simulink model "ExampleTransformation"  (R2024a)
settings: Solver=FixedStepAuto  StartTime=0.0  StopTime=inf  FixedStep=0.02  RelTol=1e-3  EnableMultiTasking=on
undefined symbols (not defined in the file): atmosphericScattering, basicProperties, castShadow, emissionColorMultiplier, meshID, position, quaternion, scale, visible
libraries: PRISMA x17, simulink_extras x3, GenericTarget x1
settings Model: Creator=damerius  LastModifiedBy=Scythe
settings SolverCC: ConcurrentTasks=on  AlgebraicLoopSolver=TrustRegion  PositivePriorityOrder=on
settings DataIOCC: SaveOutput=off  SignalLogging=off  DSMLogging=off  SaveTime=off  ReturnWorkspaceOutputs=off
settings OptimizationCC: DefaultParameterBehavior=Inlined  ReuseModelBlockBuffer=off  ZeroExternalMemoryAtStartup=off  ZeroInternalMemoryAtStartup=off  SimCompilerOptimization=on
settings DebuggingCC: UnconnectedInputMsg=warning  UnconnectedOutputMsg=warning  UnconnectedLineMsg=warning
settings HardwareCC: ProdBitPerLong=64  ProdHWDeviceType=Intel->x86-64 (Linux 64)
settings ModelReferenceCC: EnableRefExpFcnMdlSchedulingChecks=on
settings SFSimCC: SimParseCustomCode=off  SimGenImportedTypeDefs=on  SimTargetLang=C++
settings RTWCC: GenCodeOnly=on  PackageGeneratedCodeAndArtifacts=on  PackageName=PackNGo  RTWVerbose=off  BuildConfiguration=Faster Runs  TargetLang=C++  GPUComputeCapability=3.5  DLArmComputeVersion=19.05
settings CodeAppCC: ForceParamTrailComments=on  MaxIdLength=95  MATLABSourceComments=on  UseSimReservedNames=on
settings GRTTargetCC: TargetLangStandard=C++11 (ISO)  GenerateFullHeader=off  MatFileLogging=off  CodeInterfacePackaging=C++ class

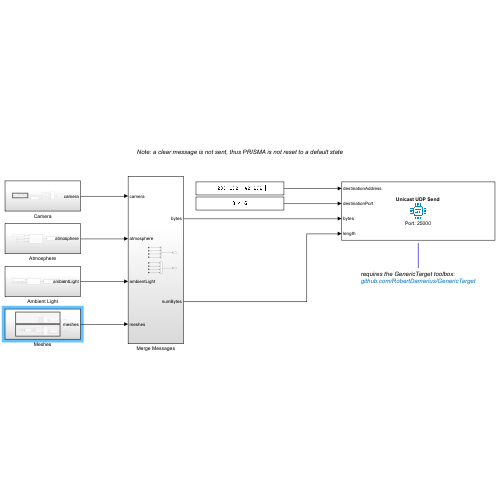
[thumbnail: Simulink's stored preview of the top-level diagram]
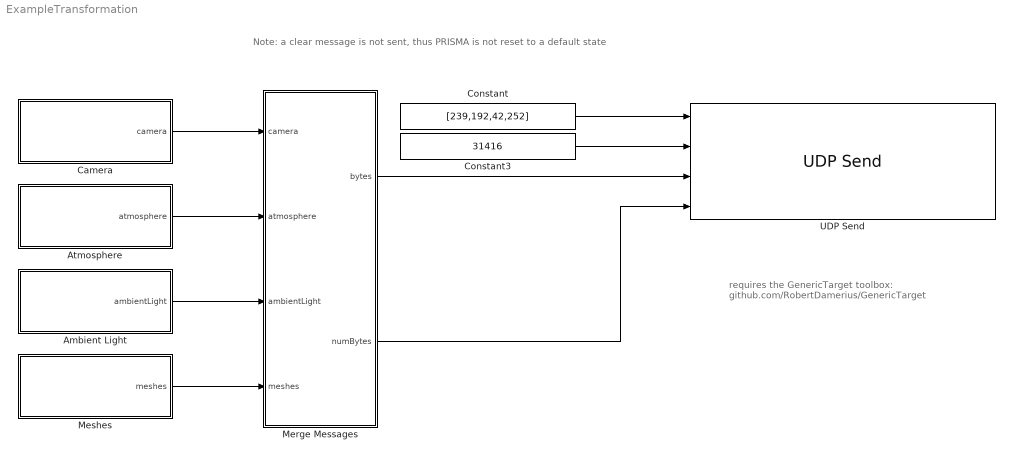
== system ExampleTransformation ==
  note: Note: a clear message is not sent, thus PRISMA is not reset to a default state
  note: requires the GenericTarget toolbox:
      | github.com/RobertDamerius/GenericTarget
  Ambient Light : Subsystem
  Atmosphere : Subsystem
  Camera : Subsystem
  Constant : Constant  Value=[239,192,42,252]  OutDataTypeStr=uint8
  Constant3 : Constant  Value=31416  OutDataTypeStr=uint16
  Merge Messages : Subsystem
  Meshes : Subsystem
  UDP Send : GenericTarget/Interface/UDP Send  showDetails=off  interfacePort=25000  interfaceIP=[0,0,0,0]  deviceName=''  prioritySocket=6  allowBroadcast=off  SampleTime=-1
      settings: SourceProductName=Generic Target
  wires:
  Constant3/1 -> UDP Send/2
  Camera/1(camera) -> Merge Messages/1(camera)
  Meshes/1(meshes) -> Merge Messages/4(meshes)
  Merge Messages/1(bytes) -> UDP Send/3
  Merge Messages/2(numBytes) -> UDP Send/4
  Ambient Light/1(ambientLight) -> Merge Messages/3(ambientLight)
  Constant/1 -> UDP Send/1
  Atmosphere/1(atmosphere) -> Merge Messages/2(atmosphere)

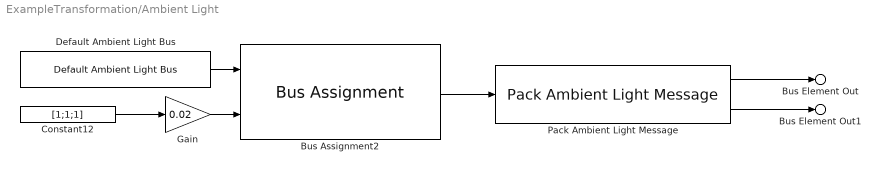
== system ExampleTransformation/Ambient Light ==
  Bus Assignment2 : BusAssignment  AssignedSignals=color
  Constant12 : Constant  Value=[1;1;1]
  Default Ambient Light Bus : PRISMA/Default Ambient Light Bus
      settings: SourceProductName=PRISMA
  Gain : Gain  Gain=0.02
  Pack Ambient Light Message : PRISMA/Pack Ambient Light Message
      settings: SourceProductName=PRISMA
  Bus Element Out : Outport  PortName=ambientLight  Element=bytes
  Bus Element Out1 : Outport  PortName=ambientLight  Element=numBytes
  wires:
  Pack Ambient Light Message/2 -> Bus Element Out1/1
  Pack Ambient Light Message/1 -> Bus Element Out/1
  Gain/1 -> Bus Assignment2/2
  Constant12/1 -> Gain/1
  Default Ambient Light Bus/1 -> Bus Assignment2/1
  Bus Assignment2/1 -> Pack Ambient Light Message/1

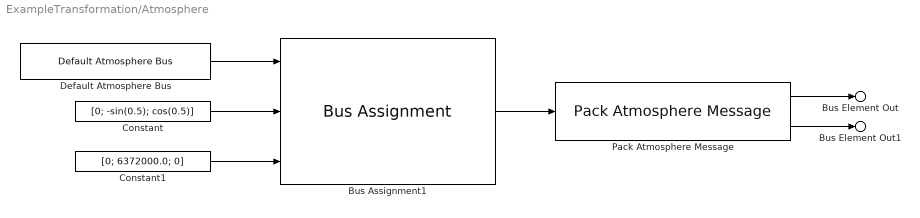
== system ExampleTransformation/Atmosphere ==
  Bus Assignment1 : BusAssignment  AssignedSignals=basicProperties.sunLightDirection,atmosphericScattering.eyePosition
  Constant : Constant  Value=[0; -sin(0.5); cos(0.5)]
  Constant1 : Constant  Value=[0; 6372000.0; 0]
  Default Atmosphere Bus : PRISMA/Default Atmosphere Bus
      settings: SourceProductName=PRISMA
  Pack Atmosphere Message : PRISMA/Pack Atmosphere Message
      settings: SourceProductName=PRISMA
  Bus Element Out : Outport  PortName=atmosphere  Element=bytes
  Bus Element Out1 : Outport  PortName=atmosphere  Element=numBytes
  wires:
  Bus Assignment1/1 -> Pack Atmosphere Message/1
  Default Atmosphere Bus/1 -> Bus Assignment1/1
  Pack Atmosphere Message/1 -> Bus Element Out/1
  Pack Atmosphere Message/2 -> Bus Element Out1/1
  Constant/1 -> Bus Assignment1/2
  Constant1/1 -> Bus Assignment1/3

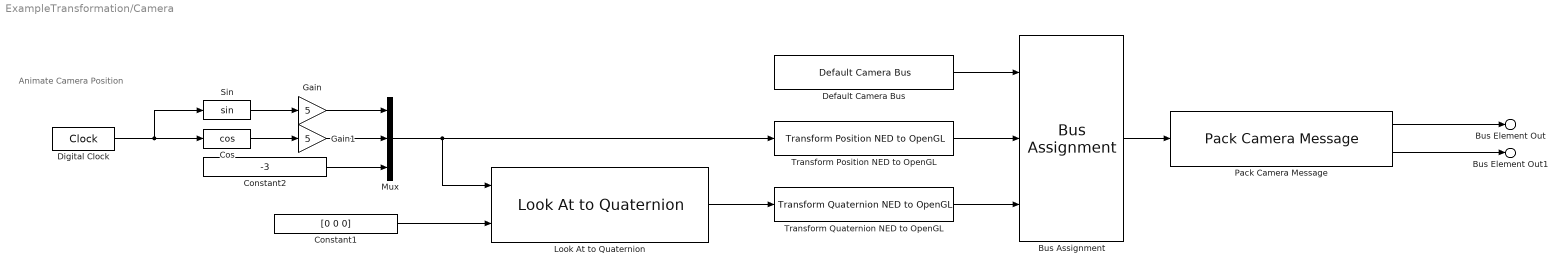
== system ExampleTransformation/Camera ==
  note: Animate Camera Position
  Bus Assignment : BusAssignment  AssignedSignals=position,quaternion
  Constant1 : Constant  Value=[0 0 0]
  Constant2 : Constant  Value=-3
  Cos : Trigonometry  Operator=cos
  Default Camera Bus : PRISMA/Default Camera Bus
      settings: SourceProductName=PRISMA
  Digital Clock : DigitalClock  SampleTime=0.02
  Gain : Gain  Gain=5
  Gain1 : Gain  Gain=5
  Look At to Quaternion : PRISMA/Transformation/Look At to Quaternion
      settings: SourceProductName=PRISMA
  Mux : Mux  Inputs=3
  Pack Camera Message : PRISMA/Pack Camera Message
      settings: SourceProductName=PRISMA
  Sin : Trigonometry
  Transform Position NED to OpenGL : PRISMA/Transformation/Transform Position NED to OpenGL
      settings: SourceProductName=PRISMA
  Transform Quaternion NED to OpenGL : PRISMA/Transformation/Transform Quaternion NED to OpenGL
      settings: SourceProductName=PRISMA
  Bus Element Out : Outport  PortName=camera  Element=bytes
  Bus Element Out1 : Outport  PortName=camera  Element=numBytes
  wires:
  Default Camera Bus/1 -> Bus Assignment/1
  Bus Assignment/1 -> Pack Camera Message/1
  Transform Position NED to OpenGL/1 -> Bus Assignment/2
  Transform Quaternion NED to OpenGL/1 -> Bus Assignment/3
  Look At to Quaternion/1 -> Transform Quaternion NED to OpenGL/1
  Mux/1 -> Look At to Quaternion/1, Transform Position NED to OpenGL/1
  Constant1/1 -> Look At to Quaternion/2
  Pack Camera Message/1 -> Bus Element Out/1
  Pack Camera Message/2 -> Bus Element Out1/1
  Constant2/1 -> Mux/3
  Sin/1 -> Gain/1
  Gain/1 -> Mux/1
  Cos/1 -> Gain1/1
  Gain1/1 -> Mux/2
  Digital Clock/1 -> Sin/1, Cos/1

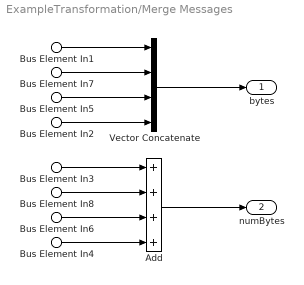
== system ExampleTransformation/Merge Messages ==
  Bus Element In1 : Inport  PortName=camera  Element=bytes
  Bus Element In3 : Inport  PortName=camera  Element=numBytes
  Bus Element In7 : Inport  Port=2  PortName=atmosphere  Element=bytes
  Bus Element In8 : Inport  Port=2  PortName=atmosphere  Element=numBytes
  Bus Element In5 : Inport  Port=3  PortName=ambientLight  Element=bytes
  Bus Element In6 : Inport  Port=3  PortName=ambientLight  Element=numBytes
  Bus Element In2 : Inport  Port=4  PortName=meshes  Element=bytes
  Bus Element In4 : Inport  Port=4  PortName=meshes  Element=numBytes
  Add : Sum  Inputs=++++
  Vector Concatenate : Concatenate  NumInputs=4
  bytes : Outport
  numBytes : Outport  Port=2
  wires:
  Bus Element In1/1 -> Vector Concatenate/1
  Bus Element In2/1 -> Vector Concatenate/4
  Bus Element In3/1 -> Add/1
  Bus Element In4/1 -> Add/4
  Vector Concatenate/1 -> bytes/1
  Add/1 -> numBytes/1
  Bus Element In5/1 -> Vector Concatenate/3
  Bus Element In6/1 -> Add/3
  Bus Element In7/1 -> Vector Concatenate/2
  Bus Element In8/1 -> Add/2

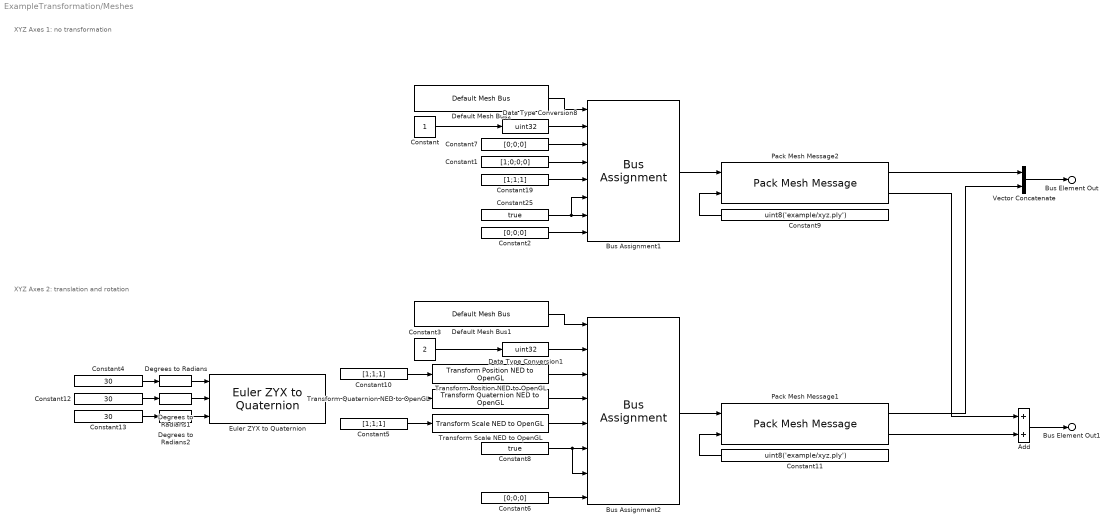
== system ExampleTransformation/Meshes ==
  note: XYZ Axes 1: no transformation
  note: XYZ Axes 2: translation and rotation
  Add : Sum
  Bus Assignment1 : BusAssignment  AssignedSignals=meshID,position,quaternion,scale,visible,castShadow,emissionColorMultiplier
  Bus Assignment2 : BusAssignment  AssignedSignals=meshID,position,quaternion,scale,visible,castShadow,emissionColorMultiplier
  Constant : Constant
  Constant1 : Constant  Value=[1;0;0;0]
  Constant10 : Constant  Value=[1;1;1]
  Constant11 : Constant  Value=uint8('example/xyz.ply')  OutDataTypeStr=uint8
  Constant12 : Constant  Value=30
  Constant13 : Constant  Value=30
  Constant19 : Constant  Value=[1;1;1]
  Constant2 : Constant  Value=[0;0;0]
  Constant25 : Constant  Value=true  OutDataTypeStr=boolean
  Constant3 : Constant  Value=2
  Constant4 : Constant  Value=30
  Constant5 : Constant  Value=[1;1;1]
  Constant6 : Constant  Value=[0;0;0]
  Constant7 : Constant  Value=[0;0;0]
  Constant8 : Constant  Value=true  OutDataTypeStr=boolean
  Constant9 : Constant  Value=uint8('example/xyz.ply')  OutDataTypeStr=uint8
  Data Type Conversion1 : DataTypeConversion  OutDataTypeStr=uint32  SaturateOnIntegerOverflow=off  RndMeth=Floor
  Data Type Conversion8 : DataTypeConversion  OutDataTypeStr=uint32  SaturateOnIntegerOverflow=off  RndMeth=Floor
  Default Mesh Bus1 : PRISMA/Default Mesh Bus
      settings: SourceProductName=PRISMA
  Default Mesh Bus2 : PRISMA/Default Mesh Bus
      settings: SourceProductName=PRISMA
  Degrees to Radians : simulink_extras/Transformations/Degrees to Radians
  Degrees to Radians1 : simulink_extras/Transformations/Degrees to Radians
  Degrees to Radians2 : simulink_extras/Transformations/Degrees to Radians
  Euler ZYX to Quaternion : PRISMA/Transformation/Euler ZYX to Quaternion
      settings: SourceProductName=PRISMA
  Pack Mesh Message1 : PRISMA/Pack Mesh Message
      settings: SourceProductName=PRISMA
  Pack Mesh Message2 : PRISMA/Pack Mesh Message
      settings: SourceProductName=PRISMA
  Transform Position NED to OpenGL : PRISMA/Transformation/Transform Position NED to OpenGL
      settings: SourceProductName=PRISMA
  Transform Quaternion NED to OpenGL : PRISMA/Transformation/Transform Quaternion NED to OpenGL
      settings: SourceProductName=PRISMA
  Transform Scale NED to OpenGL : PRISMA/Transformation/Transform Scale NED to OpenGL
      settings: SourceProductName=PRISMA
  Vector Concatenate : Concatenate
  Bus Element Out : Outport  PortName=meshes  Element=bytes
  Bus Element Out1 : Outport  PortName=meshes  Element=numBytes
  wires:
  Euler ZYX to Quaternion/1 -> Transform Quaternion NED to OpenGL/1
  Transform Quaternion NED to OpenGL/1 -> Bus Assignment2/4
  Transform Scale NED to OpenGL/1 -> Bus Assignment2/5
  Constant10/1 -> Transform Position NED to OpenGL/1
  Constant5/1 -> Transform Scale NED to OpenGL/1
  Transform Position NED to OpenGL/1 -> Bus Assignment2/3
  Constant13/1 -> Degrees to Radians2/1
  Constant12/1 -> Degrees to Radians1/1
  Degrees to Radians2/1 -> Euler ZYX to Quaternion/3
  Degrees to Radians1/1 -> Euler ZYX to Quaternion/2
  Degrees to Radians/1 -> Euler ZYX to Quaternion/1
  Constant4/1 -> Degrees to Radians/1
  Constant11/1 -> Pack Mesh Message1/2
  Default Mesh Bus1/1 -> Bus Assignment2/1
  Bus Assignment2/1 -> Pack Mesh Message1/1
  Data Type Conversion1/1 -> Bus Assignment2/2
  Constant8/1 -> Bus Assignment2/6, Bus Assignment2/7
  Constant3/1 -> Data Type Conversion1/1
  Constant6/1 -> Bus Assignment2/8
  Constant2/1 -> Bus Assignment1/8
  Constant/1 -> Data Type Conversion8/1
  Constant1/1 -> Bus Assignment1/4
  Constant7/1 -> Bus Assignment1/3
  Constant25/1 -> Bus Assignment1/7, Bus Assignment1/6
  Data Type Conversion8/1 -> Bus Assignment1/2
  Bus Assignment1/1 -> Pack Mesh Message2/1
  Constant19/1 -> Bus Assignment1/5
  Default Mesh Bus2/1 -> Bus Assignment1/1
  Constant9/1 -> Pack Mesh Message2/2
  Pack Mesh Message2/1 -> Vector Concatenate/1
  Pack Mesh Message1/1 -> Vector Concatenate/2
  Vector Concatenate/1 -> Bus Element Out/1
  Pack Mesh Message1/2 -> Add/2
  Pack Mesh Message2/2 -> Add/1
  Add/1 -> Bus Element Out1/1
